simulink model "sim_IL_H2DF_2024a"  (R2024a)
settings: Solver=FixedStepAuto  StartTime=0.0  StopTime=4899  FixedStep=1  RelTol=1e-3  EnableMultiTasking=on
model workspace (MAT data in the model file):
  enable_IMEP_noise = 100
  enable_IMEP_offset = 1
values from neighbouring files (symbols this model uses):
  IL = struct()    [init_simulink_IL_H2DF.m]
undefined symbols (not defined in the file or in its folder): C2C_NMPC, cost_length, horizon_length, y_ref_buf
libraries: dspswit3 x4, deeplib x1
(part 1 of 2)
settings Model: ExtModeTrigDuration=2  Creator=maxim  LastModifiedBy=winkler_a
settings SolverCC: PositivePriorityOrder=on
settings OptimizationCC: EnhancedBackFolding=on  PassReuseOutputArgsAs=Individual arguments  ZeroExternalMemoryAtStartup=off  ZeroInternalMemoryAtStartup=off  MaxStackSize=64  OptimizeBlockOrder=speed  DifferentSizesBufferReuse=on  OptimizationCustomize=off  EfficientTunableParamExpr=on
settings DebuggingCC: ParameterTunabilityLossMsg=error
settings HardwareCC: ProdBitPerPointer=32  ProdBitPerSizeT=32  ProdBitPerPtrDiffT=32  ProdLargestAtomicInteger=Long  ProdLargestAtomicFloat=Double  ProdWordSize=32  ProdLongLongMode=on  ProdHWDeviceType=ARM Compatible->ARM Cortex
settings RTWCC: Description=Embedded Coder  SystemTargetFile=ert.tlc  HardwareBoard=Raspberry Pi  TLCOptions="-aInlineSetEventsForThisBaseRateFcn=TLC_FALSE -aSuppressMultiTaskScheduler=TLC_FALSE  -aRateBasedStepFcn=0"  TemplateMakefile=ert_default_tmf  GenerateReport=on  RTWUseSimCustomCode=on  Toolchain=GNU GCC Embedded Linux  BuildConfiguration=Faster Runs  CodeExecutionProfiling=on  GPUComputeCapability=3.5
settings CodeAppCC: ForceParamTrailComments=on  IgnoreCustomStorageClasses=off  OperatorAnnotations=on  SimulinkDataObjDesc=on  SFDataObjDesc=on  InsertBlockDesc=on
settings ERTTargetCC: SupportContinuousTime=on  SupportNonInlinedSFcns=on  SupportVariableSizeSignals=on

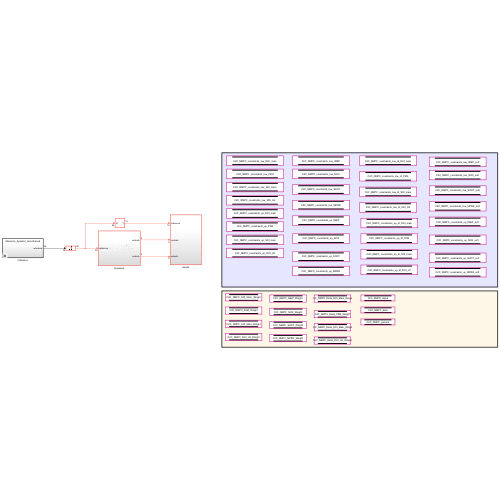
[thumbnail: Simulink's stored preview of the top-level diagram]
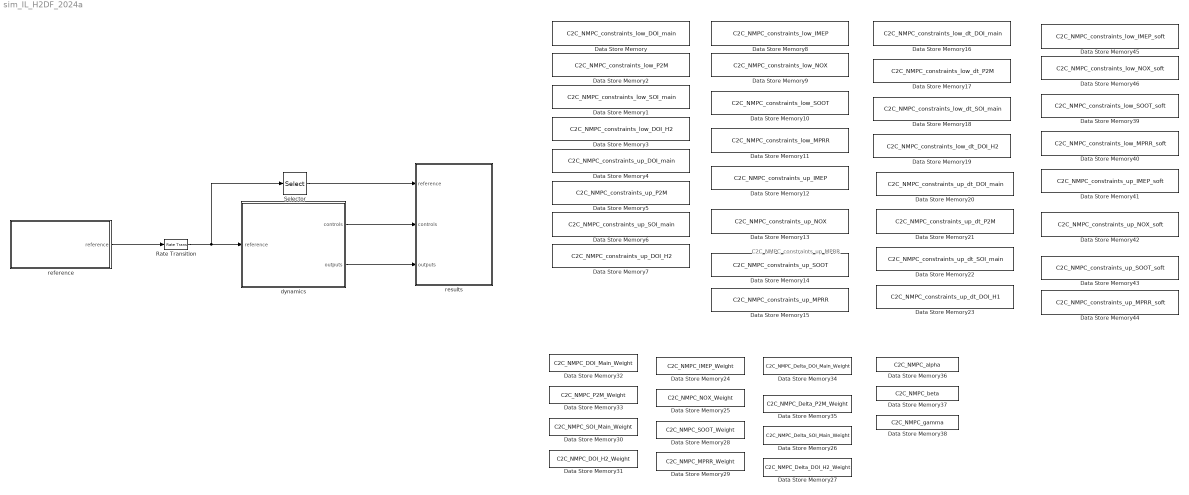
== system sim_IL_H2DF_2024a ==
  note: C2C_NMPC_constraints_up_MPRR
  Data Store Memory : DataStoreMemory  DataStoreName=C2C_NMPC_constraints_low_DOI_main  WriteAfterWriteMsg=warning  ShowAdditionalParam=off
  Data Store Memory1 : DataStoreMemory  DataStoreName=C2C_NMPC_constraints_low_SOI_main  WriteAfterWriteMsg=warning  ShowAdditionalParam=off
  Data Store Memory10 : DataStoreMemory  DataStoreName=C2C_NMPC_constraints_low_SOOT  WriteAfterWriteMsg=warning  ShowAdditionalParam=off
  Data Store Memory11 : DataStoreMemory  DataStoreName=C2C_NMPC_constraints_low_MPRR  WriteAfterWriteMsg=warning  ShowAdditionalParam=off
  Data Store Memory12 : DataStoreMemory  DataStoreName=C2C_NMPC_constraints_up_IMEP  WriteAfterWriteMsg=warning  ShowAdditionalParam=off
  Data Store Memory13 : DataStoreMemory  DataStoreName=C2C_NMPC_constraints_up_NOX  WriteAfterWriteMsg=warning  ShowAdditionalParam=off
  Data Store Memory14 : DataStoreMemory  DataStoreName=C2C_NMPC_constraints_up_SOOT  WriteAfterWriteMsg=warning  ShowAdditionalParam=off
  Data Store Memory15 : DataStoreMemory  DataStoreName=C2C_NMPC_constraints_up_MPRR  WriteAfterWriteMsg=warning  ShowAdditionalParam=off
  Data Store Memory16 : DataStoreMemory  DataStoreName=C2C_NMPC_constraints_low_dt_DOI_main  WriteAfterWriteMsg=warning  ShowAdditionalParam=off
  Data Store Memory17 : DataStoreMemory  DataStoreName=C2C_NMPC_constraints_low_dt_P2M  WriteAfterWriteMsg=warning  ShowAdditionalParam=off
  Data Store Memory18 : DataStoreMemory  DataStoreName=C2C_NMPC_constraints_low_dt_SOI_main  WriteAfterWriteMsg=warning  ShowAdditionalParam=off
  Data Store Memory19 : DataStoreMemory  DataStoreName=C2C_NMPC_constraints_low_dt_DOI_H2  WriteAfterWriteMsg=warning  ShowAdditionalParam=off
  Data Store Memory2 : DataStoreMemory  DataStoreName=C2C_NMPC_constraints_low_P2M  WriteAfterWriteMsg=warning  ShowAdditionalParam=off
  Data Store Memory20 : DataStoreMemory  DataStoreName=C2C_NMPC_constraints_up_dt_DOI_main  WriteAfterWriteMsg=warning  ShowAdditionalParam=off
  Data Store Memory21 : DataStoreMemory  DataStoreName=C2C_NMPC_constraints_up_dt_P2M  WriteAfterWriteMsg=warning  ShowAdditionalParam=off
  Data Store Memory22 : DataStoreMemory  DataStoreName=C2C_NMPC_constraints_up_dt_SOI_main  WriteAfterWriteMsg=warning  ShowAdditionalParam=off
  Data Store Memory23 : DataStoreMemory  DataStoreName=C2C_NMPC_constraints_up_dt_DOI_H1  WriteAfterWriteMsg=warning  ShowAdditionalParam=off
  Data Store Memory24 : DataStoreMemory  DataStoreName=C2C_NMPC_IMEP_Weight  WriteAfterWriteMsg=warning  ShowAdditionalParam=off
  Data Store Memory25 : DataStoreMemory  DataStoreName=C2C_NMPC_NOX_Weight  WriteAfterWriteMsg=warning  ShowAdditionalParam=off
  Data Store Memory26 : DataStoreMemory  DataStoreName=C2C_NMPC_Delta_SOI_Main_Weight  WriteAfterWriteMsg=warning  ShowAdditionalParam=off
  Data Store Memory27 : DataStoreMemory  DataStoreName=C2C_NMPC_Delta_DOI_H2_Weight  WriteAfterWriteMsg=warning  ShowAdditionalParam=off
  Data Store Memory28 : DataStoreMemory  DataStoreName=C2C_NMPC_SOOT_Weight  WriteAfterWriteMsg=warning  ShowAdditionalParam=off
  Data Store Memory29 : DataStoreMemory  DataStoreName=C2C_NMPC_MPRR_Weight  WriteAfterWriteMsg=warning  ShowAdditionalParam=off
  Data Store Memory3 : DataStoreMemory  DataStoreName=C2C_NMPC_constraints_low_DOI_H2  WriteAfterWriteMsg=warning  ShowAdditionalParam=off
  Data Store Memory30 : DataStoreMemory  DataStoreName=C2C_NMPC_SOI_Main_Weight  WriteAfterWriteMsg=warning  ShowAdditionalParam=off
  Data Store Memory31 : DataStoreMemory  DataStoreName=C2C_NMPC_DOI_H2_Weight  WriteAfterWriteMsg=warning  ShowAdditionalParam=off
  Data Store Memory32 : DataStoreMemory  DataStoreName=C2C_NMPC_DOI_Main_Weight  WriteAfterWriteMsg=warning  ShowAdditionalParam=off
  Data Store Memory33 : DataStoreMemory  DataStoreName=C2C_NMPC_P2M_Weight  WriteAfterWriteMsg=warning  ShowAdditionalParam=off
  Data Store Memory34 : DataStoreMemory  DataStoreName=C2C_NMPC_Delta_DOI_Main_Weight  WriteAfterWriteMsg=warning  ShowAdditionalParam=off
  Data Store Memory35 : DataStoreMemory  DataStoreName=C2C_NMPC_Delta_P2M_Weight  WriteAfterWriteMsg=warning  ShowAdditionalParam=off
  Data Store Memory36 : DataStoreMemory  DataStoreName=C2C_NMPC_alpha  WriteAfterWriteMsg=warning  ShowAdditionalParam=off
  Data Store Memory37 : DataStoreMemory  DataStoreName=C2C_NMPC_beta  WriteAfterWriteMsg=warning  ShowAdditionalParam=off
  Data Store Memory38 : DataStoreMemory  DataStoreName=C2C_NMPC_gamma  WriteAfterWriteMsg=warning  ShowAdditionalParam=off
  Data Store Memory39 : DataStoreMemory  DataStoreName=C2C_NMPC_constraints_low_SOOT_soft  WriteAfterWriteMsg=warning  ShowAdditionalParam=off
  Data Store Memory4 : DataStoreMemory  DataStoreName=C2C_NMPC_constraints_up_DOI_main  WriteAfterWriteMsg=warning  ShowAdditionalParam=off
  Data Store Memory40 : DataStoreMemory  DataStoreName=C2C_NMPC_constraints_low_MPRR_soft  WriteAfterWriteMsg=warning  ShowAdditionalParam=off
  Data Store Memory41 : DataStoreMemory  DataStoreName=C2C_NMPC_constraints_up_IMEP_soft  WriteAfterWriteMsg=warning  ShowAdditionalParam=off
  Data Store Memory42 : DataStoreMemory  DataStoreName=C2C_NMPC_constraints_up_NOX_soft  WriteAfterWriteMsg=warning  ShowAdditionalParam=off
  Data Store Memory43 : DataStoreMemory  DataStoreName=C2C_NMPC_constraints_up_SOOT_soft  WriteAfterWriteMsg=warning  ShowAdditionalParam=off
  Data Store Memory44 : DataStoreMemory  DataStoreName=C2C_NMPC_constraints_up_MPRR_soft  WriteAfterWriteMsg=warning  ShowAdditionalParam=off
  Data Store Memory45 : DataStoreMemory  DataStoreName=C2C_NMPC_constraints_low_IMEP_soft  WriteAfterWriteMsg=warning  ShowAdditionalParam=off
  Data Store Memory46 : DataStoreMemory  DataStoreName=C2C_NMPC_constraints_low_NOX_soft  WriteAfterWriteMsg=warning  ShowAdditionalParam=off
  Data Store Memory5 : DataStoreMemory  DataStoreName=C2C_NMPC_constraints_up_P2M  WriteAfterWriteMsg=warning  ShowAdditionalParam=off
  Data Store Memory6 : DataStoreMemory  DataStoreName=C2C_NMPC_constraints_up_SOI_main  WriteAfterWriteMsg=warning  ShowAdditionalParam=off
  Data Store Memory7 : DataStoreMemory  DataStoreName=C2C_NMPC_constraints_up_DOI_H2  WriteAfterWriteMsg=warning  ShowAdditionalParam=off
  Data Store Memory8 : DataStoreMemory  DataStoreName=C2C_NMPC_constraints_low_IMEP  WriteAfterWriteMsg=warning  ShowAdditionalParam=off
  Data Store Memory9 : DataStoreMemory  DataStoreName=C2C_NMPC_constraints_low_NOX  WriteAfterWriteMsg=warning  ShowAdditionalParam=off
  Rate Transition : RateTransition  Integrity=off  OutPortSampleTime=1
  Selector : Selector  InputPortWidth=C2C_NMPC.Dims.n_cost*3  IndexOptions=Index vector (dialog)  Indices=1:C2C_NMPC.Dims.n_cost  OutputSizes=1
  dynamics : Subsystem
  reference : Subsystem  Variant=on  VariantControlMode=label  VariantControl=Choice  LabelModeActiveChoice=reference_dynamic_smoothened_steps_msmtn
  results : Subsystem
  wires:
  dynamics/2(outputs) -> results/3(outputs)
  Rate Transition/1 -> dynamics/1(reference), Selector/1
  dynamics/1(controls) -> results/2(controls)
  Selector/1 -> results/1(reference)
  reference/1(reference) -> Rate Transition/1

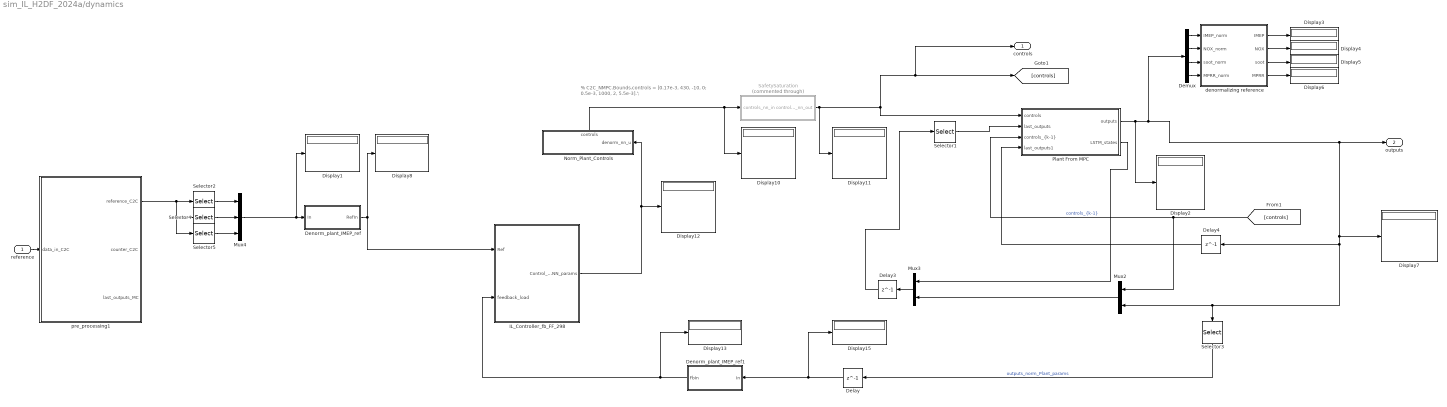
== system sim_IL_H2DF_2024a/dynamics ==
  note: % C2C_NMPC.Bounds.controls = [0.17e-3, 430, -10, 0;
      | 							0.5e-3, 1000, 2, 5.5e-3].';
  reference : Inport
  Delay : Delay  DelayLength=1  InitialCondition=0
  Delay3 : Delay  DelayLength=1  InitialCondition=C2C_NMPC.x0
  Delay4 : Delay  DelayLength=1  InitialCondition=C2C_NMPC.x0((C2C_NMPC.Dims.n_states - C2C_NMPC.Dims.n_outputs + 1):C2C_NMPC.Dims.n_states)
  Demux : Demux
  Denorm_plant_IMEP_ref : Subsystem
  Denorm_plant_IMEP_ref1 : Subsystem
  Display{1..8,10..13,15} (13 alike) : Display
  IL_Controller_fb_FF_298 : Subsystem  VariantControl=fb_LSTM_321_syn
  Mux2 : Mux  Inputs=2
  Mux3 : Mux  Inputs=2
  Mux4 : Mux  Inputs=3
  Norm_Plant_Controls : Subsystem
      settings: PortSchema="{\"entries\":[{\"content\":{\"sides\":[{\"content\":{\"connectorIds\":[\"In1\"]},\"type\":\"ConnectorPlacement.EquallySpacedRectSide\",\"uuid\":\"dacbf39b-836c-4129-b483-c12a7b9212cd\"},{\"content\":{\"side\":\"RIGHT\"},\"type\":\"ConnectorPlacement.EquallySpacedRectSide\",\"uuid\":\"2d78ef8c-cdc0-4bce-ac21-e70953625460\"},{\"content\":{\"connectorIds\":[\"Out1\"],\"side\":\"TOP\"},\"type\":\"ConnectorPlacement.EquallySpacedRectSide\",\"uuid\":\"db73efac-16fa-4395-b9f0-b65c608dd2b1\"}]},\"type\":\"ConnectorPlacement.EquallySpacedConnector\",\"uuid\":\"80b02a92-2029-43df-9a0c-0ef0e755e1ed\"}],\"packageUris\":[\"http://schema.mathworks.com/mf0/Connector/R2020b\"],\"version\":\"1.0\"}"
  Plant From MPC : Subsystem  Variant=on  VariantControlMode=label  VariantControl=Choice  LabelModeActiveChoice=Choice
  SafetySaturation : Subsystem  Commented=through
  Selector1 : Selector  IndexOptions=Index vector (dialog)  Indices=[(C2C_NMPC.Dims.n_states - C2C_NMPC.Dims.n_outputs + 1):C2C_NMPC.Dims.n_states]  OutputSizes=1
  Selector2 : Selector  IndexOptions=Index vector (dialog)  Indices=5  OutputSizes=1
  Selector3 : Selector  IndexOptions=Index vector (dialog)  Indices=[1]  OutputSizes=1
  Selector4 : Selector  IndexOptions=Index vector (dialog)  Indices=[ (C2C_NMPC.Dims.n_cost + 5) : (C2C_NMPC.Dims.n_cost + 5) ]  OutputSizes=1
  Selector5 : Selector  IndexOptions=Index vector (dialog)  Indices=[ (C2C_NMPC.Dims.n_cost * 2 + 5) : (C2C_NMPC.Dims.n_cost * 2 + 5 ) ]  OutputSizes=1
  denormalizing reference : Subsystem
  pre_processing1 : Subsystem
  controls : Outport
  outputs : Outport  Port=2
  wires:
  Delay3/1 -> Selector1/1
  Mux3/1 -> Delay3/1
  Mux2/1 -> Mux3/2
  reference/1 -> pre_processing1/1(data_in_C2C)
  Plant From MPC/1(outputs) -> outputs/1, Delay4/1, Selector3/1, Mux2/2, Display7/1, Demux/1, Display2/1
  Demux/2 -> denormalizing reference/2(NOX_norm)
  Demux/1 -> denormalizing reference/1(IMEP_norm)
  Demux/3 -> denormalizing reference/3(soot_norm)
  Demux/4 -> denormalizing reference/4(MPRR_norm)
  denormalizing reference/1(IMEP) -> Display3/1
  denormalizing reference/4(MPRR) -> Display6/1
  denormalizing reference/3(soot) -> Display5/1
  denormalizing reference/2(NOX) -> Display4/1
  IL_Controller_fb_FF_298/1(Control_norm_NN_params) -> Norm_Plant_Controls/1(denorm_nn_u), Display12/1
  Delay/1 -> Denorm_plant_IMEP_ref1/1(In), Display15/1
  Selector3/1 -> Delay/1  "outputs_norm_Plant_params"
  [controls] -> Plant From MPC/3("controls_{k-1}"), Mux2/1  "controls_{k-1}"
  Mux4/1 -> Display1/1, Denorm_plant_IMEP_ref/1(In)
  Selector2/1 -> Mux4/1
  Selector4/1 -> Mux4/2
  Selector5/1 -> Mux4/3
  pre_processing1/1(reference_C2C) -> Selector2/1, Selector4/1, Selector5/1
  Denorm_plant_IMEP_ref/1(RefIn) -> IL_Controller_fb_FF_298/1(Ref), Display8/1
  Denorm_plant_IMEP_ref1/1(FbIn) -> IL_Controller_fb_FF_298/2(feedback_load), Display13/1
  Norm_Plant_Controls/1(controls) -> Display10/1, SafetySaturation/1(controls_nn_in)
  Selector1/1 -> Plant From MPC/2(last_outputs)
  Delay4/1 -> Plant From MPC/4(last_outputs1)
  Plant From MPC/2(LSTM_states) -> Mux3/1
  SafetySaturation/1(controls_nn_out) -> Display11/1, Plant From MPC/1(controls), controls/1, [controls]

== system sim_IL_H2DF_2024a/reference ==
  note: ref is hardcoded for N=3 now
  reference_dynamic : Subsystem  Variant=on  VariantControlMode=label  VariantControl=reference_dynamic_steps  LabelModeActiveChoice=Choice_1
  reference_dynamic_constant : Subsystem  Variant=on  VariantControlMode=label  VariantControl=reference_dynamic_constant  LabelModeActiveChoice=Choice_1
  reference_dynamic_random_steps : Subsystem  Variant=on  VariantControlMode=label  VariantControl=reference_dynamic_steps_random  LabelModeActiveChoice=Choice_1
  reference_dynamic_smoothened : Subsystem  Variant=on  VariantControlMode=label  VariantControl=reference_dynamic_smoothened_steps_msmtn  LabelModeActiveChoice=Choice_1
  reference_dynamic_smoothened_random_fast_steps : Subsystem  Variant=on  VariantControlMode=label  VariantControl=reference_dynamic_smoothened_fast_steps_random  LabelModeActiveChoice=Choice_1
  reference_dynamic_smoothened_random_slow_steps : Subsystem  Variant=on  VariantControlMode=label  VariantControl=reference_dynamic_smoothened_slow_steps_random  LabelModeActiveChoice=Choice_1
  reference_static : Subsystem  VariantControl=reference_static
  reference : Outport

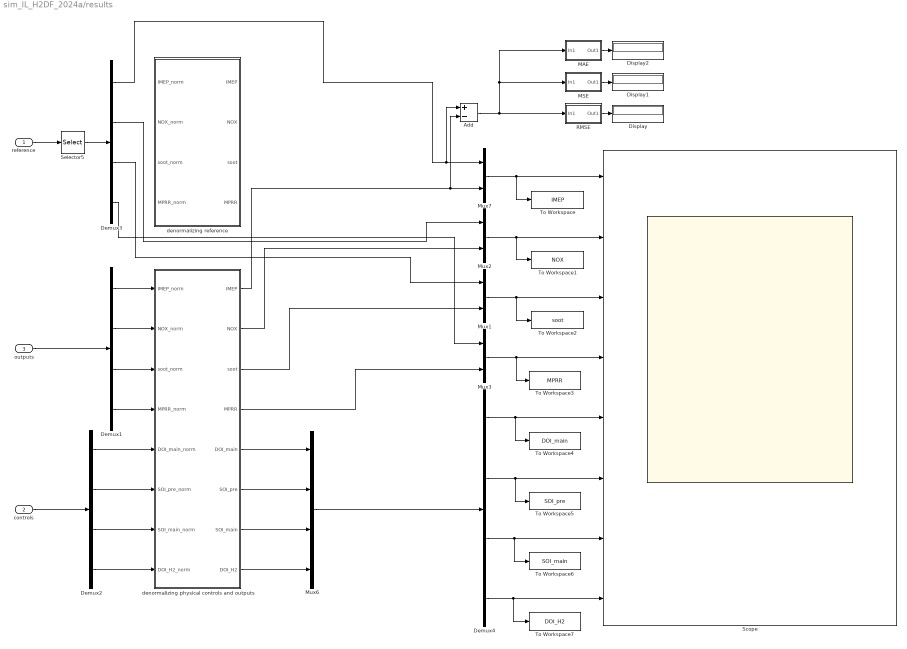
== system sim_IL_H2DF_2024a/results ==
  reference : Inport
  controls : Inport  Port=2
  outputs : Inport  Port=3
  Add : Sum  Inputs=+-
  Demux{1..4} (4 alike) : Demux
  Display : Display
  Display1 : Display
  Display2 : Display
  MAE : Subsystem
  MSE : Subsystem
  Mux{1..3,7} (4 alike) : Mux  Inputs=2
  Mux6 : Mux
  RMSE : Subsystem
  Scope : Scope  NumInputPorts=8
  Selector5 : Selector  IndexOptions=Index vector (dialog)  Indices=[(C2C_NMPC.Dims.n_controls + 1 ):(C2C_NMPC.Dims.n_cost - C2C_NMPC.Dims.n_controls)]  OutputSizes=1
  To Workspace : ToWorkspace  VariableName=IMEP  SampleTime=-1
  To Workspace1 : ToWorkspace  VariableName=NOX  SampleTime=-1
  To Workspace2 : ToWorkspace  VariableName=soot  SampleTime=-1
  To Workspace3 : ToWorkspace  VariableName=MPRR  SampleTime=-1
  To Workspace4 : ToWorkspace  VariableName=DOI_main  SampleTime=-1
  To Workspace5 : ToWorkspace  VariableName=SOI_pre  SampleTime=-1
  To Workspace6 : ToWorkspace  VariableName=SOI_main  SampleTime=-1
  To Workspace7 : ToWorkspace  VariableName=DOI_H2  SampleTime=-1
  denormalizing physical controls and outputs : Subsystem
  denormalizing reference : Subsystem
  wires:
  reference/1 -> Selector5/1
  Selector5/1 -> Demux3/1
  outputs/1 -> Demux1/1
  controls/1 -> Demux2/1
  Mux7/1 -> To Workspace/1, Scope/1
  Mux2/1 -> To Workspace1/1, Scope/2
  Demux3/1 -> Mux7/1, Add/1
  Mux3/1 -> To Workspace3/1, Scope/4
  Mux1/1 -> To Workspace2/1, Scope/3
  Demux4/2 -> To Workspace5/1, Scope/6
  Demux4/3 -> To Workspace6/1, Scope/7
  Demux4/1 -> To Workspace4/1, Scope/5
  Mux6/1 -> Demux4/1
  Demux1/1 -> denormalizing physical controls and outputs/1(IMEP_norm)
  Demux1/2 -> denormalizing physical controls and outputs/2(NOX_norm)
  Demux1/3 -> denormalizing physical controls and outputs/3(soot_norm)
  Demux1/4 -> denormalizing physical controls and outputs/4(MPRR_norm)
  Demux2/1 -> denormalizing physical controls and outputs/5(DOI_main_norm)
  Demux2/2 -> denormalizing physical controls and outputs/6(SOI_pre_norm)
  Demux2/3 -> denormalizing physical controls and outputs/7(SOI_main_norm)
  denormalizing physical controls and outputs/1(IMEP) -> Add/2, Mux7/2
  denormalizing physical controls and outputs/5(DOI_main) -> Mux6/1
  denormalizing physical controls and outputs/6(SOI_pre) -> Mux6/2
  denormalizing physical controls and outputs/7(SOI_main) -> Mux6/3
  Demux3/3 -> Mux1/1
  Demux3/4 -> Mux3/1
  denormalizing physical controls and outputs/2(NOX) -> Mux2/2
  denormalizing physical controls and outputs/3(soot) -> Mux1/2
  denormalizing physical controls and outputs/4(MPRR) -> Mux3/2
  Demux2/4 -> denormalizing physical controls and outputs/8(DOI_H2_norm)
  denormalizing physical controls and outputs/8(DOI_H2) -> Mux6/4
  Demux4/4 -> To Workspace7/1, Scope/8
  Demux3/2 -> Mux2/1
  Add/1 -> MAE/1(In1), MSE/1(In1), RMSE/1(In1)
  RMSE/1(Out1) -> Display/1
  MSE/1(Out1) -> Display1/1
  MAE/1(Out1) -> Display2/1

== system sim_IL_H2DF_2024a/dynamics/Denorm_plant_IMEP_ref ==
  In : Inport
  Constant : Constant  Value=C2C_NMPC.Normalization.outputs.mean(1)
  Gain : Gain  Gain=C2C_NMPC.Normalization.outputs.std(1)
  Sum6 : Sum  Inputs=|++
  RefIn : Outport
  wires:
  In/1 -> Gain/1  "IMEP"
  Sum6/1 -> RefIn/1
  Gain/1 -> Sum6/1
  Constant/1 -> Sum6/2

== system sim_IL_H2DF_2024a/dynamics/Denorm_plant_IMEP_ref1 ==
  In : Inport
  Constant : Constant  Value=C2C_NMPC.Normalization.outputs.mean(1)
  Gain : Gain  Gain=C2C_NMPC.Normalization.outputs.std(1)
  Sum6 : Sum  Inputs=|++
  FbIn : Outport
  wires:
  In/1 -> Gain/1  "IMEP"
  Sum6/1 -> FbIn/1
  Gain/1 -> Sum6/1
  Constant/1 -> Sum6/2

== system sim_IL_H2DF_2024a/dynamics/IL_Controller_fb_FF_298 ==
  Ref : Inport
  feedback_load : Inport  Port=2
  Data Type Conversion : DataTypeConversion  OutDataTypeStr=double  SaturateOnIntegerOverflow=off  RndMeth=Floor
  Denorm_NN_Controls : Subsystem
  Mux : Mux  Inputs=2
  Norm_NN_IMEP_ref : Subsystem
  Norm_NN_IMEP_ref1 : Subsystem
  Predict : deeplib/Predict  Network=Network from MAT-file  NetworkFunction=squeezenet  NetworkFilePath=h2df_model_2024_0012_0008_0298.mat  MiniBatchSize=512  InputDataFormats={'',''}  Predictions=on  Activations={}  ForceInterpretedSim=off  EnableDLNetwork=on  LastKnownNetworkFilePath=''  LastKnownNetworkTimeStamp=''
  Control_norm_NN_params : Outport
  wires:
  Ref/1 -> Norm_NN_IMEP_ref/1(In)
  Data Type Conversion/1 -> Denorm_NN_Controls/1(controls_nn)  "Control_norm_NN_params"
  Mux/1 -> Predict/1
  Norm_NN_IMEP_ref/1(Out) -> Mux/1
  Norm_NN_IMEP_ref1/1(Out) -> Mux/2
  Denorm_NN_Controls/1(denorm_nn_u) -> Control_norm_NN_params/1
  feedback_load/1 -> Norm_NN_IMEP_ref1/1(In)
  Predict/1 -> Data Type Conversion/1

== system sim_IL_H2DF_2024a/dynamics/Norm_Plant_Controls ==
  denorm_nn_u : Inport
  Constant10 : Constant  Value=C2C_NMPC.Normalization.controls.mean(2)
  Constant11 : Constant  Value=C2C_NMPC.Normalization.controls.mean(3)
  Constant12 : Constant  Value=C2C_NMPC.Normalization.controls.mean(4)
  Constant9 : Constant  Value=C2C_NMPC.Normalization.controls.mean(1)
  Demux : Demux
  Gain4 : Gain  Gain=1/C2C_NMPC.Normalization.controls.std(1)
  Gain5 : Gain  Gain=1/C2C_NMPC.Normalization.controls.std(2)
  Gain6 : Gain  Gain=1/C2C_NMPC.Normalization.controls.std(3)
  Gain7 : Gain  Gain=1/C2C_NMPC.Normalization.controls.std(4)
  Mux1 : Mux
  Sum{4,6..8} (4 alike) : Sum  Inputs=|+-
  controls : Outport
  wires:
  Mux1/1 -> controls/1
  denorm_nn_u/1 -> Demux/1
  Sum8/1 -> Gain7/1
  Demux/3 -> Sum7/1  "SOI_main"
  Constant12/1 -> Sum8/2
  Sum7/1 -> Gain6/1
  Constant11/1 -> Sum7/2
  Gain5/1 -> Mux1/2
  Gain4/1 -> Mux1/1
  Gain7/1 -> Mux1/4
  Demux/1 -> Sum4/1  "DOI_main"
  Constant9/1 -> Sum4/2
  Demux/2 -> Sum6/1  "SOI_pre"
  Sum4/1 -> Gain4/1
  Gain6/1 -> Mux1/3
  Constant10/1 -> Sum6/2
  Demux/4 -> Sum8/1  "DOI_H2"
  Sum6/1 -> Gain5/1

== system sim_IL_H2DF_2024a/dynamics/Plant From MPC ==
  controls : Inport
  last_outputs : Inport  Port=2
  "controls_{k-1}" : Inport  Port=3
  last_outputs1 : Inport  Port=4
  Hardcoded : Subsystem  VariantControl=Choice
  outputs : Outport
  LSTM_states : Outport  Port=2

== system sim_IL_H2DF_2024a/dynamics/SafetySaturation ==
  controls_nn_in : Inport
  Demux : Demux
  Mux : Mux
  Saturation : Saturate  UpperLimit=C2C_NMPC.Bounds.controls_norm(1,2)  LowerLimit=C2C_NMPC.Bounds.controls_norm(1,1)
  Saturation1 : Saturate  UpperLimit=C2C_NMPC.Bounds.controls_norm(2,2)  LowerLimit=C2C_NMPC.Bounds.controls_norm(2,1)
  Saturation2 : Saturate  UpperLimit=C2C_NMPC.Bounds.controls_norm(3,2)  LowerLimit=C2C_NMPC.Bounds.controls_norm(3,1)
  Saturation3 : Saturate  UpperLimit=C2C_NMPC.Bounds.controls_norm(4,2)  LowerLimit=C2C_NMPC.Bounds.controls_norm(4,1)
  controls_nn_out : Outport
  wires:
  controls_nn_in/1 -> Demux/1
  Demux/1 -> Saturation/1
  Demux/2 -> Saturation1/1
  Demux/3 -> Saturation2/1
  Demux/4 -> Saturation3/1
  Mux/1 -> controls_nn_out/1
  Saturation/1 -> Mux/1
  Saturation1/1 -> Mux/2
  Saturation2/1 -> Mux/3
  Saturation3/1 -> Mux/4

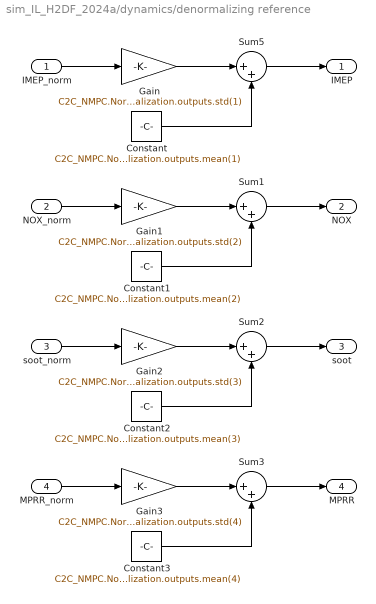
== system sim_IL_H2DF_2024a/dynamics/denormalizing reference ==
  IMEP_norm : Inport
  NOX_norm : Inport  Port=2
  soot_norm : Inport  Port=3
  MPRR_norm : Inport  Port=4
  Constant : Constant  Value=C2C_NMPC.Normalization.outputs.mean(1)
  Constant1 : Constant  Value=C2C_NMPC.Normalization.outputs.mean(2)
  Constant2 : Constant  Value=C2C_NMPC.Normalization.outputs.mean(3)
  Constant3 : Constant  Value=C2C_NMPC.Normalization.outputs.mean(4)
  Gain : Gain  Gain=C2C_NMPC.Normalization.outputs.std(1)
  Gain1 : Gain  Gain=C2C_NMPC.Normalization.outputs.std(2)
  Gain2 : Gain  Gain=C2C_NMPC.Normalization.outputs.std(3)
  Gain3 : Gain  Gain=C2C_NMPC.Normalization.outputs.std(4)
  Sum{1..3,5} (4 alike) : Sum  Inputs=|++
  IMEP : Outport
  NOX : Outport  Port=2
  soot : Outport  Port=3
  MPRR : Outport  Port=4
  wires:
  Gain/1 -> Sum5/1
  IMEP_norm/1 -> Gain/1
  Constant/1 -> Sum5/2
  Sum5/1 -> IMEP/1
  Gain1/1 -> Sum1/1
  Constant1/1 -> Sum1/2
  NOX_norm/1 -> Gain1/1
  Sum1/1 -> NOX/1
  Gain2/1 -> Sum2/1
  Constant2/1 -> Sum2/2
  soot_norm/1 -> Gain2/1
  Sum2/1 -> soot/1
  Gain3/1 -> Sum3/1
  Constant3/1 -> Sum3/2
  MPRR_norm/1 -> Gain3/1
  Sum3/1 -> MPRR/1

== system sim_IL_H2DF_2024a/dynamics/pre_processing1 ==
  data_in_C2C : Inport
  Selector : Selector  IndexOptions=Index vector (dialog)  Indices=[6]  OutputSizes=1
  normalize_last_outputs_MC : Subsystem
  normalize_reference_C2C : Subsystem
  reference_C2C : Outport  VectorParamsAs1DForOutWhenUnconnected=off
  counter_C2C : Outport  Port=2  VectorParamsAs1DForOutWhenUnconnected=off
  last_outputs_MC : Outport  Port=3  VectorParamsAs1DForOutWhenUnconnected=off
  wires:
  Selector/1 -> counter_C2C/1
  normalize_last_outputs_MC/1(last_outputs_MC) -> last_outputs_MC/1
  data_in_C2C/1 -> normalize_reference_C2C/1(data_in), normalize_last_outputs_MC/1(data_in), Selector/1
  normalize_reference_C2C/1(reference_C2C) -> reference_C2C/1

== system sim_IL_H2DF_2024a/reference/reference_dynamic ==
  reference_dynamic : Subsystem  VariantControl=Choice_1
  reference : Outport

== system sim_IL_H2DF_2024a/reference/reference_dynamic_constant ==
  reference_dynamic_constant : Subsystem  VariantControl=Choice_1
  reference : Outport

== system sim_IL_H2DF_2024a/reference/reference_dynamic_random_steps ==
  reference_dynamic_smoothened_random : Subsystem  VariantControl=Choice_1
  reference : Outport

== system sim_IL_H2DF_2024a/reference/reference_dynamic_smoothened ==
  reference_dynamic_smoothened : Subsystem  VariantControl=Choice_1
  reference : Outport

== system sim_IL_H2DF_2024a/reference/reference_dynamic_smoothened_random_fast_steps ==
  reference_dynamic_smoothened_random : Subsystem  VariantControl=Choice_1
  reference : Outport

== system sim_IL_H2DF_2024a/reference/reference_dynamic_smoothened_random_slow_steps ==
  reference_dynamic_smoothened_random : Subsystem  VariantControl=Choice_1
  reference : Outport

== system sim_IL_H2DF_2024a/reference/reference_static ==
  Add1 : Sum
  Clock : Clock
  Constant : Constant
  Constant1 : Constant  Value=[C2C_NMPC.controls_ref;C2C_NMPC.outputs_ref; zeros(C2C_NMPC.Dims.n_controls, length(C2C_NMPC.controls_ref(1, :)))]
  Mux : Mux  Inputs=3
  ref_func : MATLAB Function  TreatAsAtomicUnit=on
  reference : Outport  VectorParamsAs1DForOutWhenUnconnected=off
  wires:
  Constant1/1 -> ref_func/1(ref_norm)
  Constant/1 -> Add1/2
  Add1/1 -> ref_func/2(init_index)
  Clock/1 -> Add1/1
  Mux/1 -> reference/1
  ref_func/1(y_ref) -> Mux/3, Mux/1, Mux/2

== system sim_IL_H2DF_2024a/results/MAE ==
  In1 : Inport
  Abs : Abs  SaturateOnIntegerOverflow=off
  Add1 : Sum
  Constant : Constant  Value=4899
  Delay : Delay  DelayLength=1
  Divide : Product  Inputs=*/
  Out1 : Outport
  wires:
  Divide/1 -> Out1/1
  Add1/1 -> Delay/1
  Delay/1 -> Divide/1, Add1/2
  Abs/1 -> Add1/1
  In1/1 -> Abs/1
  Constant/1 -> Divide/2

== system sim_IL_H2DF_2024a/results/MSE ==
  In1 : Inport
  Add1 : Sum
  Constant : Constant  Value=4899
  Delay : Delay  DelayLength=1
  Divide : Product  Inputs=*/
  Square : Math  Operator=square
  Out1 : Outport
  wires:
  Divide/1 -> Out1/1
  Add1/1 -> Delay/1
  Delay/1 -> Divide/1, Add1/2
  Square/1 -> Add1/1
  In1/1 -> Square/1
  Constant/1 -> Divide/2

== system sim_IL_H2DF_2024a/results/RMSE ==
  In1 : Inport
  Add1 : Sum
  Constant : Constant  Value=4899
  Delay : Delay  DelayLength=1
  Divide : Product  Inputs=*/
  Sqrt : Sqrt
  Square : Math  Operator=square
  Out1 : Outport
  wires:
  Sqrt/1 -> Out1/1
  Add1/1 -> Delay/1
  Delay/1 -> Divide/1, Add1/2
  Square/1 -> Add1/1
  Divide/1 -> Sqrt/1
  In1/1 -> Square/1
  Constant/1 -> Divide/2

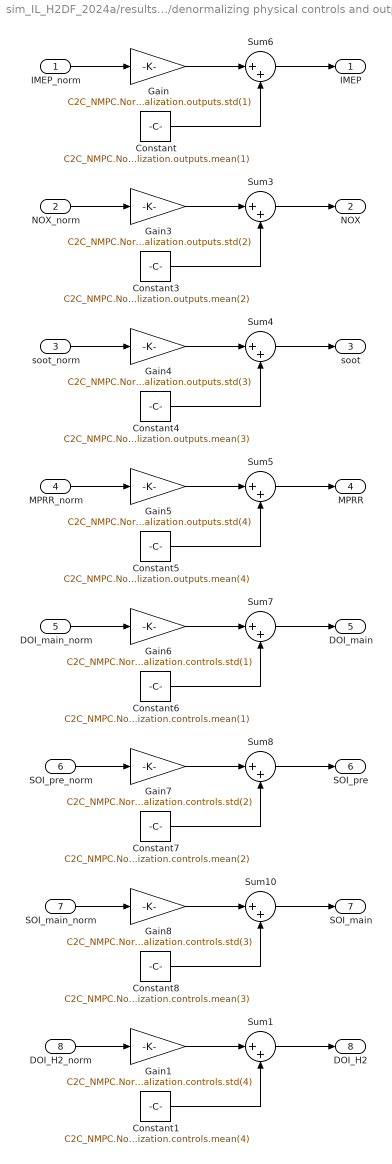
== system sim_IL_H2DF_2024a/results/denormalizing physical controls and outputs ==
  IMEP_norm : Inport
  NOX_norm : Inport  Port=2
  soot_norm : Inport  Port=3
  MPRR_norm : Inport  Port=4
  DOI_main_norm : Inport  Port=5
  SOI_pre_norm : Inport  Port=6
  SOI_main_norm : Inport  Port=7
  DOI_H2_norm : Inport  Port=8
  Constant : Constant  Value=C2C_NMPC.Normalization.outputs.mean(1)
  Constant1 : Constant  Value=C2C_NMPC.Normalization.controls.mean(4)
  Constant3 : Constant  Value=C2C_NMPC.Normalization.outputs.mean(2)
  Constant4 : Constant  Value=C2C_NMPC.Normalization.outputs.mean(3)
  Constant5 : Constant  Value=C2C_NMPC.Normalization.outputs.mean(4)
  Constant6 : Constant  Value=C2C_NMPC.Normalization.controls.mean(1)
  Constant7 : Constant  Value=C2C_NMPC.Normalization.controls.mean(2)
  Constant8 : Constant  Value=C2C_NMPC.Normalization.controls.mean(3)
  Gain : Gain  Gain=C2C_NMPC.Normalization.outputs.std(1)
  Gain1 : Gain  Gain=C2C_NMPC.Normalization.controls.std(4)
  Gain3 : Gain  Gain=C2C_NMPC.Normalization.outputs.std(2)
  Gain4 : Gain  Gain=C2C_NMPC.Normalization.outputs.std(3)
  Gain5 : Gain  Gain=C2C_NMPC.Normalization.outputs.std(4)
  Gain6 : Gain  Gain=C2C_NMPC.Normalization.controls.std(1)
  Gain7 : Gain  Gain=C2C_NMPC.Normalization.controls.std(2)
  Gain8 : Gain  Gain=C2C_NMPC.Normalization.controls.std(3)
  Sum{1,3..8,10} (8 alike) : Sum  Inputs=|++
  IMEP : Outport
  NOX : Outport  Port=2
  soot : Outport  Port=3
  MPRR : Outport  Port=4
  DOI_main : Outport  Port=5
  SOI_pre : Outport  Port=6
  SOI_main : Outport  Port=7
  DOI_H2 : Outport  Port=8
  wires:
  Gain4/1 -> Sum4/1
  Constant3/1 -> Sum3/2
  Constant4/1 -> Sum4/2
  Gain3/1 -> Sum3/1
  Constant5/1 -> Sum5/2
  Gain5/1 -> Sum5/1
  Constant/1 -> Sum6/2
  Sum3/1 -> NOX/1
  NOX_norm/1 -> Gain3/1
  Sum5/1 -> MPRR/1
  Gain/1 -> Sum6/1
  IMEP_norm/1 -> Gain/1
  Sum6/1 -> IMEP/1
  MPRR_norm/1 -> Gain5/1
  Sum4/1 -> soot/1
  soot_norm/1 -> Gain4/1
  Constant7/1 -> Sum8/2
  Gain8/1 -> Sum10/1
  Constant6/1 -> Sum7/2
  Gain7/1 -> Sum8/1
  Sum10/1 -> SOI_main/1
  DOI_main_norm/1 -> Gain6/1
  Sum7/1 -> DOI_main/1
  Gain6/1 -> Sum7/1
  Sum8/1 -> SOI_pre/1
  Constant8/1 -> Sum10/2
  SOI_main_norm/1 -> Gain8/1
  SOI_pre_norm/1 -> Gain7/1
  DOI_H2_norm/1 -> Gain1/1
  Constant1/1 -> Sum1/2
  Gain1/1 -> Sum1/1
  Sum1/1 -> DOI_H2/1

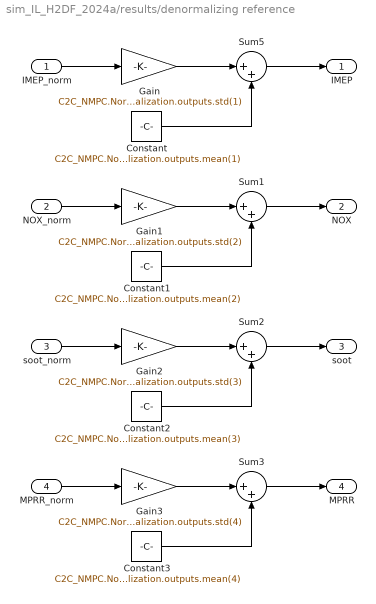
== system sim_IL_H2DF_2024a/results/denormalizing reference ==
  IMEP_norm : Inport
  NOX_norm : Inport  Port=2
  soot_norm : Inport  Port=3
  MPRR_norm : Inport  Port=4
  Constant : Constant  Value=C2C_NMPC.Normalization.outputs.mean(1)
  Constant1 : Constant  Value=C2C_NMPC.Normalization.outputs.mean(2)
  Constant2 : Constant  Value=C2C_NMPC.Normalization.outputs.mean(3)
  Constant3 : Constant  Value=C2C_NMPC.Normalization.outputs.mean(4)
  Gain : Gain  Gain=C2C_NMPC.Normalization.outputs.std(1)
  Gain1 : Gain  Gain=C2C_NMPC.Normalization.outputs.std(2)
  Gain2 : Gain  Gain=C2C_NMPC.Normalization.outputs.std(3)
  Gain3 : Gain  Gain=C2C_NMPC.Normalization.outputs.std(4)
  Sum{1..3,5} (4 alike) : Sum  Inputs=|++
  IMEP : Outport
  NOX : Outport  Port=2
  soot : Outport  Port=3
  MPRR : Outport  Port=4
  wires:
  Gain/1 -> Sum5/1
  IMEP_norm/1 -> Gain/1
  Constant/1 -> Sum5/2
  Sum5/1 -> IMEP/1
  Gain1/1 -> Sum1/1
  Constant1/1 -> Sum1/2
  NOX_norm/1 -> Gain1/1
  Sum1/1 -> NOX/1
  Gain2/1 -> Sum2/1
  Constant2/1 -> Sum2/2
  soot_norm/1 -> Gain2/1
  Sum2/1 -> soot/1
  Gain3/1 -> Sum3/1
  Constant3/1 -> Sum3/2
  MPRR_norm/1 -> Gain3/1
  Sum3/1 -> MPRR/1

== system sim_IL_H2DF_2024a/dynamics/IL_Controller_fb_FF_298/Denorm_NN_Controls ==
  controls_nn : Inport
  Constant4 : Constant  Value=IL.Normalization.outputs.mean(1)
  Constant5 : Constant  Value=IL.Normalization.outputs.mean(2)
  Constant6 : Constant  Value=IL.Normalization.outputs.mean(3)
  Constant7 : Constant  Value=IL.Normalization.outputs.mean(4)
  Demux : Demux
  Gain4 : Gain  Gain=IL.Normalization.outputs.std(1)
  Gain5 : Gain  Gain=IL.Normalization.outputs.std(2)
  Gain6 : Gain  Gain=IL.Normalization.outputs.std(3)
  Gain7 : Gain  Gain=IL.Normalization.outputs.std(4)
  Mux : Mux
  Sum{4,6..8} (4 alike) : Sum  Inputs=|++
  denorm_nn_u : Outport
  wires:
  Sum4/1 -> Mux/2
  Sum6/1 -> Mux/3
  controls_nn/1 -> Demux/1
  Demux/2 -> Gain5/1  "P2M"
  Demux/3 -> Gain6/1  "SOI_main"
  Demux/4 -> Gain7/1  "DOI_H2"
  Demux/1 -> Gain4/1  "DOI_main"
  Mux/1 -> denorm_nn_u/1
  Gain7/1 -> Sum7/1
  Gain6/1 -> Sum6/1
  Constant7/1 -> Sum7/2
  Constant5/1 -> Sum4/2
  Gain4/1 -> Sum8/1
  Gain5/1 -> Sum4/1
  Constant6/1 -> Sum6/2
  Constant4/1 -> Sum8/2
  Sum8/1 -> Mux/1
  Sum7/1 -> Mux/4

== system sim_IL_H2DF_2024a/dynamics/IL_Controller_fb_FF_298/Norm_NN_IMEP_ref ==
  In : Inport
  Constant9 : Constant  Value=IL.Normalization.inputs.mean(1)
  Gain4 : Gain  Gain=1/IL.Normalization.inputs.std(1)
  Sum4 : Sum  Inputs=|+-
  Out : Outport
  wires:
  In/1 -> Sum4/1  "IMEP"
  Constant9/1 -> Sum4/2
  Sum4/1 -> Gain4/1
  Gain4/1 -> Out/1

== system sim_IL_H2DF_2024a/dynamics/IL_Controller_fb_FF_298/Norm_NN_IMEP_ref1 ==
  In : Inport
  Constant9 : Constant  Value=IL.Normalization.inputs.mean(1)
  Gain4 : Gain  Gain=1/IL.Normalization.inputs.std(1)
  Sum4 : Sum  Inputs=|+-
  Out : Outport
  wires:
  Gain4/1 -> Out/1
  Sum4/1 -> Gain4/1
  Constant9/1 -> Sum4/2
  In/1 -> Sum4/1  "IMEP"

== system sim_IL_H2DF_2024a/dynamics/Plant From MPC/Hardcoded ==
  controls : Inport
  last_outputs : Inport  Port=2
  "controls_{k-1}" : Inport  Port=3
  last_outputs1 : Inport  Port=4
  Delay2 : Delay  DelayLength=1  InitialCondition=C2C_NMPC.x0(1:C2C_NMPC.Dims.n_LSTM_states)
  dyn_H2DF : Subsystem  Variant=on  VariantControlMode=label  VariantControl=Choice  LabelModeActiveChoice=dyn_H2DF
  dyn_H2DF_state_augmentation : Subsystem  Variant=on  VariantControlMode=label  VariantControl=Choice  LabelModeActiveChoice=dyn_H2DF
  outputs : Outport
  LSTM_states : Outport  Port=2
  wires:
  Delay2/1 -> dyn_H2DF_state_augmentation/1(last_LSTM_states), dyn_H2DF/3(last_LSTM_states)
  last_outputs/1 -> dyn_H2DF/2(last_outputs)
  dyn_H2DF_state_augmentation/1(LSTM_states) -> LSTM_states/1, Delay2/1
  controls/1 -> dyn_H2DF/1(controls)
  dyn_H2DF/1(outputs) -> outputs/1
  "controls_{k-1}"/1 -> dyn_H2DF_state_augmentation/2(controls)
  last_outputs1/1 -> dyn_H2DF_state_augmentation/3(last_outputs)

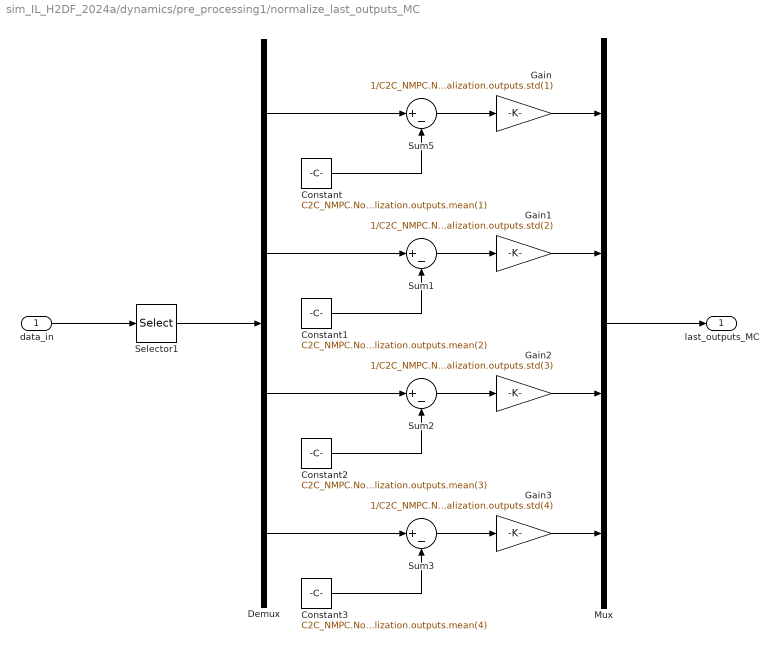
== system sim_IL_H2DF_2024a/dynamics/pre_processing1/normalize_last_outputs_MC ==
  data_in : Inport
  Constant : Constant  Value=C2C_NMPC.Normalization.outputs.mean(1)
  Constant1 : Constant  Value=C2C_NMPC.Normalization.outputs.mean(2)
  Constant2 : Constant  Value=C2C_NMPC.Normalization.outputs.mean(3)
  Constant3 : Constant  Value=C2C_NMPC.Normalization.outputs.mean(4)
  Demux : Demux
  Gain : Gain  Gain=1/C2C_NMPC.Normalization.outputs.std(1)
  Gain1 : Gain  Gain=1/C2C_NMPC.Normalization.outputs.std(2)
  Gain2 : Gain  Gain=1/C2C_NMPC.Normalization.outputs.std(3)
  Gain3 : Gain  Gain=1/C2C_NMPC.Normalization.outputs.std(4)
  Mux : Mux
  Selector1 : Selector  IndexOptions=Index vector (dialog)  Indices=[1:4]  OutputSizes=1
  Sum{1..3,5} (4 alike) : Sum  Inputs=|+-
  last_outputs_MC : Outport  VectorParamsAs1DForOutWhenUnconnected=off
  wires:
  Selector1/1 -> Demux/1
  Demux/4 -> Sum3/1
  data_in/1 -> Selector1/1
  Demux/1 -> Sum5/1
  Constant/1 -> Sum5/2
  Sum5/1 -> Gain/1
  Gain/1 -> Mux/1
  Sum3/1 -> Gain3/1
  Constant3/1 -> Sum3/2
  Mux/1 -> last_outputs_MC/1
  Gain2/1 -> Mux/3
  Demux/3 -> Sum2/1
  Constant1/1 -> Sum1/2
  Gain1/1 -> Mux/2
  Gain3/1 -> Mux/4
  Sum1/1 -> Gain1/1
  Sum2/1 -> Gain2/1
  Constant2/1 -> Sum2/2
  Demux/2 -> Sum1/1

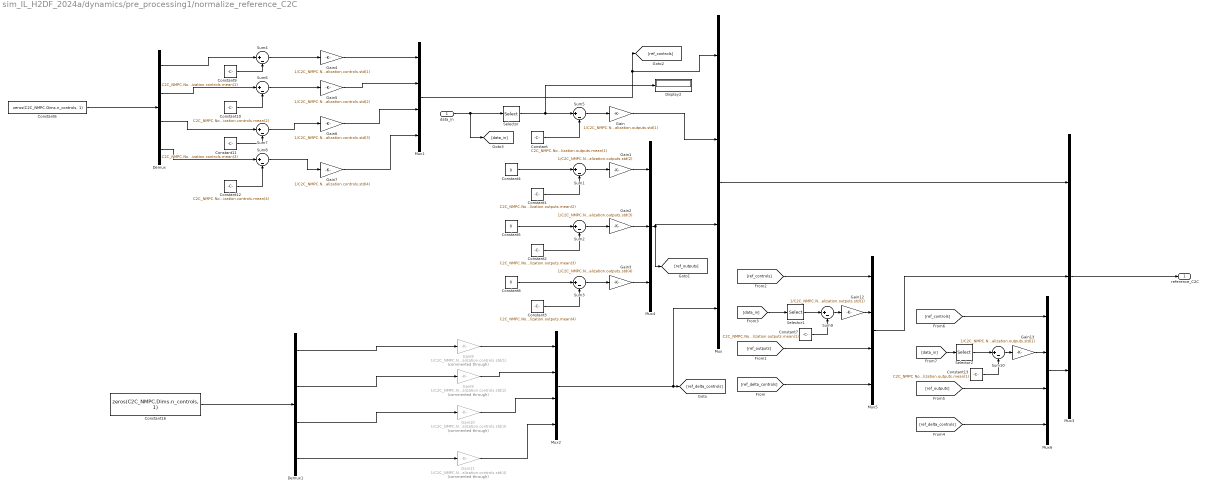
== system sim_IL_H2DF_2024a/dynamics/pre_processing1/normalize_reference_C2C ==
  data_in : Inport
  Constant : Constant  Value=C2C_NMPC.Normalization.outputs.mean(1)
  Constant1 : Constant  Value=C2C_NMPC.Normalization.outputs.mean(2)
  Constant10 : Constant  Value=C2C_NMPC.Normalization.controls.mean(2)
  Constant11 : Constant  Value=C2C_NMPC.Normalization.controls.mean(3)
  Constant12 : Constant  Value=C2C_NMPC.Normalization.controls.mean(4)
  Constant13 : Constant  Value=C2C_NMPC.Normalization.outputs.mean(1)
  Constant16 : Constant  Value=zeros(C2C_NMPC.Dims.n_controls, 1)
  Constant2 : Constant  Value=C2C_NMPC.Normalization.outputs.mean(3)
  Constant3 : Constant  Value=C2C_NMPC.Normalization.outputs.mean(4)
  Constant4 : Constant  Value=0
  Constant5 : Constant  Value=0
  Constant6 : Constant  Value=zeros(C2C_NMPC.Dims.n_controls, 1)
  Constant7 : Constant  Value=C2C_NMPC.Normalization.outputs.mean(1)
  Constant8 : Constant  Value=0
  Constant9 : Constant  Value=C2C_NMPC.Normalization.controls.mean(1)
  Demux : Demux
  Demux1 : Demux
  Display2 : Display
  Gain : Gain  Gain=1/C2C_NMPC.Normalization.outputs.std(1)
  Gain1 : Gain  Gain=1/C2C_NMPC.Normalization.outputs.std(2)
  Gain10 : Gain  Commented=through  Gain=1/C2C_NMPC.Normalization.controls.std(3)
  Gain11 : Gain  Commented=through  Gain=1/C2C_NMPC.Normalization.controls.std(4)
  Gain12 : Gain  Gain=1/C2C_NMPC.Normalization.outputs.std(1)
  Gain13 : Gain  Gain=1/C2C_NMPC.Normalization.outputs.std(1)
  Gain2 : Gain  Gain=1/C2C_NMPC.Normalization.outputs.std(3)
  Gain3 : Gain  Gain=1/C2C_NMPC.Normalization.outputs.std(4)
  Gain4 : Gain  Gain=1/C2C_NMPC.Normalization.controls.std(1)
  Gain5 : Gain  Gain=1/C2C_NMPC.Normalization.controls.std(2)
  Gain6 : Gain  Gain=1/C2C_NMPC.Normalization.controls.std(3)
  Gain7 : Gain  Gain=1/C2C_NMPC.Normalization.controls.std(4)
  Gain8 : Gain  Commented=through  Gain=1/C2C_NMPC.Normalization.controls.std(1)
  Gain9 : Gain  Commented=through  Gain=1/C2C_NMPC.Normalization.controls.std(2)
  Mux{,1..2,5..6} (5 alike) : Mux
  Mux3 : Mux  Inputs=3
  Mux4 : Mux  Inputs=3
  Selector : Selector  IndexOptions=Index vector (dialog)  Indices=[5]  OutputSizes=1
  Selector1 : Selector  IndexOptions=Index vector (dialog)  Indices=[C2C_NMPC.Dims.n_cost+5]  OutputSizes=1
  Selector2 : Selector  IndexOptions=Index vector (dialog)  Indices=[(C2C_NMPC.Dims.n_cost*2)+5]  OutputSizes=1
  Sum{1..10} (10 alike) : Sum  Inputs=|+-
  reference_C2C : Outport  VectorParamsAs1DForOutWhenUnconnected=off
  wires:
  Gain13/1 -> Mux6/2
  Selector2/1 -> Sum10/1
  Sum10/1 -> Gain13/1
  Constant13/1 -> Sum10/2
  Gain12/1 -> Mux5/2
  Constant7/1 -> Sum9/2
  Sum9/1 -> Gain12/1
  Selector1/1 -> Sum9/1
  Mux6/1 -> Mux3/3
  [ref_delta_controls] -> Mux6/4
  [ref_outputs] -> Mux6/3
  [ref_controls] -> Mux6/1
  [data_in] -> Selector2/1
  Mux5/1 -> Mux3/2
  [data_in] -> Selector1/1
  [ref_controls] -> Mux5/1
  Mux1/1 -> Mux/1, [ref_controls]
  [ref_outputs] -> Mux5/3
  [ref_delta_controls] -> Mux5/4
  Mux4/1 -> [ref_outputs], Mux/3
  Gain/1 -> Mux/2
  Gain3/1 -> Mux4/3
  Gain2/1 -> Mux4/2
  Gain1/1 -> Mux4/1
  Mux/1 -> Mux3/1
  Mux3/1 -> reference_C2C/1
  Mux2/1 -> Mux/4, [ref_delta_controls]
  Demux1/1 -> Gain8/1
  Demux1/2 -> Gain9/1
  Demux1/3 -> Gain10/1
  Demux1/4 -> Gain11/1
  Gain10/1 -> Mux2/3
  Gain8/1 -> Mux2/1
  Constant16/1 -> Demux1/1
  Gain11/1 -> Mux2/4
  Gain9/1 -> Mux2/2
  Gain6/1 -> Mux1/3
  Gain7/1 -> Mux1/4
  Demux/4 -> Sum8/1
  Sum8/1 -> Gain7/1
  Constant12/1 -> Sum8/2
  Demux/3 -> Sum7/1
  Constant11/1 -> Sum7/2
  Sum7/1 -> Gain6/1
  Gain4/1 -> Mux1/1
  Gain5/1 -> Mux1/2
  Sum6/1 -> Gain5/1
  Constant10/1 -> Sum6/2
  Demux/2 -> Sum6/1
  Constant6/1 -> Demux/1
  Constant9/1 -> Sum4/2
  Sum4/1 -> Gain4/1
  Demux/1 -> Sum4/1
  Constant3/1 -> Sum3/2
  Sum3/1 -> Gain3/1
  Constant8/1 -> Sum3/1
  Constant2/1 -> Sum2/2
  Sum2/1 -> Gain2/1
  Constant5/1 -> Sum2/1
  Constant1/1 -> Sum1/2
  Sum1/1 -> Gain1/1
  Constant4/1 -> Sum1/1
  Selector/1 -> Sum5/1, Display2/1
  Sum5/1 -> Gain/1
  data_in/1 -> Selector/1, [data_in]
  Constant/1 -> Sum5/2

== system sim_IL_H2DF_2024a/reference/reference_dynamic/reference_dynamic ==
  note: 1 -4: 0
      | 5: IMEP_ref0
      | 6 - 12: 0
      |
      | 13 - 17: 0
      | 18: IMEP_ref0
      | 19 - 24: 0
      |
      | 25 - 29: 0
      | 5: IMEP_ref0
      | 6 - 12: 0
  note: init of delays = 4 bar!
  Add1 : Sum
  Clock : Clock
  Constant : Constant
  Constant1 : Constant  Value=[C2C_NMPC.controls_ref;C2C_NMPC.outputs_ref; zeros(C2C_NMPC.Dims.n_controls, length(C2C_NMPC.controls_ref(1, :)))]
  Constant2 : Constant  Commented=on  Value=zeros(4,1)
  Constant3 : Constant  Commented=on  Value=zeros(7,1)
  Counter : dspswit3/Counter  Commented=on  Direction=Up  CountEvent=Free running  CounterSize=16 bits  MaxCount=255  InitialCount=0  Output=Count and Hit  HitValue=32  ResetInput=on  SamplesPerFrame=1  Ts=-1  CntDtype=double  HitDtype=Logical
  Delay : Delay  Commented=on  DelayLength=1
  Delay1 : Delay  Commented=on  DelayLength=1  InitialCondition=4
  Delay2 : Delay  Commented=on  InitialCondition=4
  Enabled Subsystem : Subsystem  Commented=on  TreatAsAtomicUnit=on
  GreaterThan : RelationalOperator  Commented=on  Operator=>  OutDataTypeStr=boolean  RndMeth=Simplest  InputSameDT=off
  Mux1 : Mux  Commented=on  Inputs=3
  Rate Limiter : RateLimiter  Commented=on  RisingSlewLimit=0.33  FallingSlewLimit=-0.33  SampleTimeMode=inherited  InitialCondition=3
  Signal Conversion : SignalConversion  Commented=on  OverrideOpt=off
  ref_func : MATLAB Function  InitFcn=|  TreatAsAtomicUnit=on
      | cost_length = C2C_NMPC.Dims.n_cost ;
      | horizon_length = 3;
      | %C2C_NMPC.Opts.N; 
      | y_ref_buf = zeros(cost_length, horizon_length);
  reference : Outport  VectorParamsAs1DForOutWhenUnconnected=off
  wires:
  Clock/1 -> Add1/1
  Add1/1 -> ref_func/2(init_index)
  Constant/1 -> Add1/2
  Constant1/1 -> ref_func/1(ref_norm)
  ref_func/1(y_ref) -> reference/1
  ? -> Rate Limiter/1
  Delay/1 -> Counter/1, Enabled Subsystem/Enable
  Enabled Subsystem/2(freq) -> GreaterThan/2
  GreaterThan/1 -> Delay/1
  Counter/1 -> GreaterThan/1
  Delay2/1 -> Mux1/2
  Enabled Subsystem/1(num) -> Delay1/1, Signal Conversion/1, Delay2/1
  Delay1/1 -> ?
  Signal Conversion/1 -> ?
  Constant2/1 -> Mux1/1
  Constant3/1 -> Mux1/3

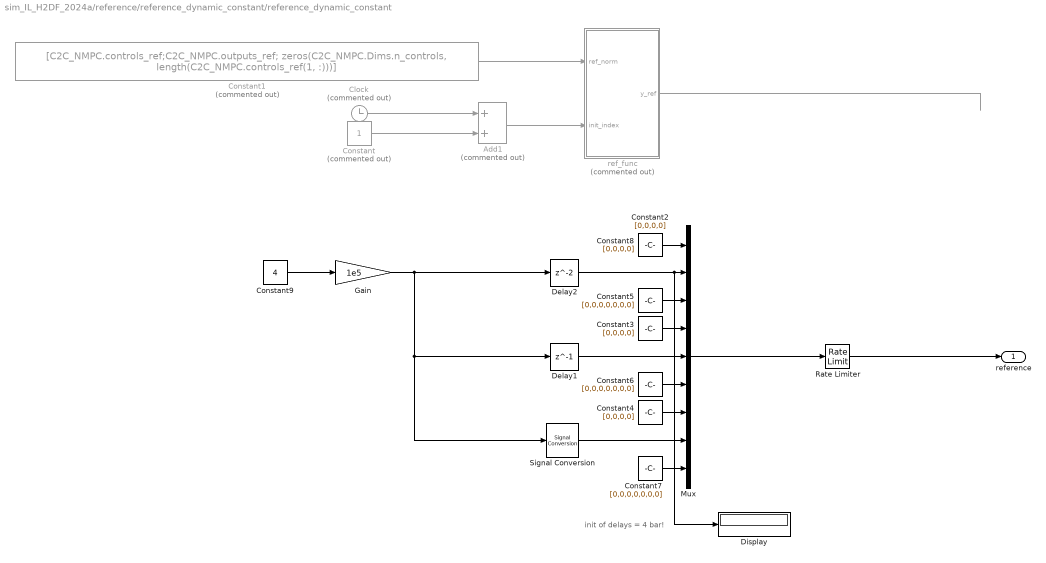
== system sim_IL_H2DF_2024a/reference/reference_dynamic_constant/reference_dynamic_constant ==
  note: init of delays = 4 bar!
  Add1 : Sum  Commented=on
  Clock : Clock  Commented=on
  Constant : Constant  Commented=on
  Constant1 : Constant  Commented=on  Value=[C2C_NMPC.controls_ref;C2C_NMPC.outputs_ref; zeros(C2C_NMPC.Dims.n_controls, length(C2C_NMPC.controls_ref(1, :)))]
  Constant{2..4,8} (4 alike) : Constant  Value=[0,0,0,0]
  Constant5 : Constant  Value=[0,0,0,0,0,0,0]
  Constant6 : Constant  Value=[0,0,0,0,0,0,0]
  Constant7 : Constant  Value=[0,0,0,0,0,0,0]
  Constant9 : Constant  Value=4
  Delay1 : Delay  DelayLength=1  InitialCondition=4
  Delay2 : Delay  InitialCondition=4
  Display : Display
  Gain : Gain  Gain=1e5
  Mux : Mux  Inputs=9
  Rate Limiter : RateLimiter  RisingSlewLimit=5000  FallingSlewLimit=-5000  SampleTimeMode=inherited  InitialCondition=3
  Signal Conversion : SignalConversion  OverrideOpt=off
  ref_func : MATLAB Function  Commented=on  InitFcn=|  TreatAsAtomicUnit=on
      | cost_length = C2C_NMPC.Dims.n_cost ;
      | horizon_length = 3;
      | %C2C_NMPC.Opts.N; 
      | y_ref_buf = zeros(cost_length, horizon_length);
  reference : Outport  VectorParamsAs1DForOutWhenUnconnected=off
  wires:
  Rate Limiter/1 -> reference/1
  Constant7/1 -> Mux/9
  Constant6/1 -> Mux/6
  Constant5/1 -> Mux/3
  Constant4/1 -> Mux/7
  Constant3/1 -> Mux/4
  Constant2/1 -> Mux/1
  Mux/1 -> Rate Limiter/1
  Delay2/1 -> Display/1, Mux/2
  Signal Conversion/1 -> Mux/8
  Constant9/1 -> Gain/1
  Delay1/1 -> Mux/5
  ref_func/1(y_ref) -> ?
  Constant1/1 -> ref_func/1(ref_norm)
  Constant/1 -> Add1/2
  Add1/1 -> ref_func/2(init_index)
  Clock/1 -> Add1/1
  Gain/1 -> Delay2/1, Delay1/1, Signal Conversion/1

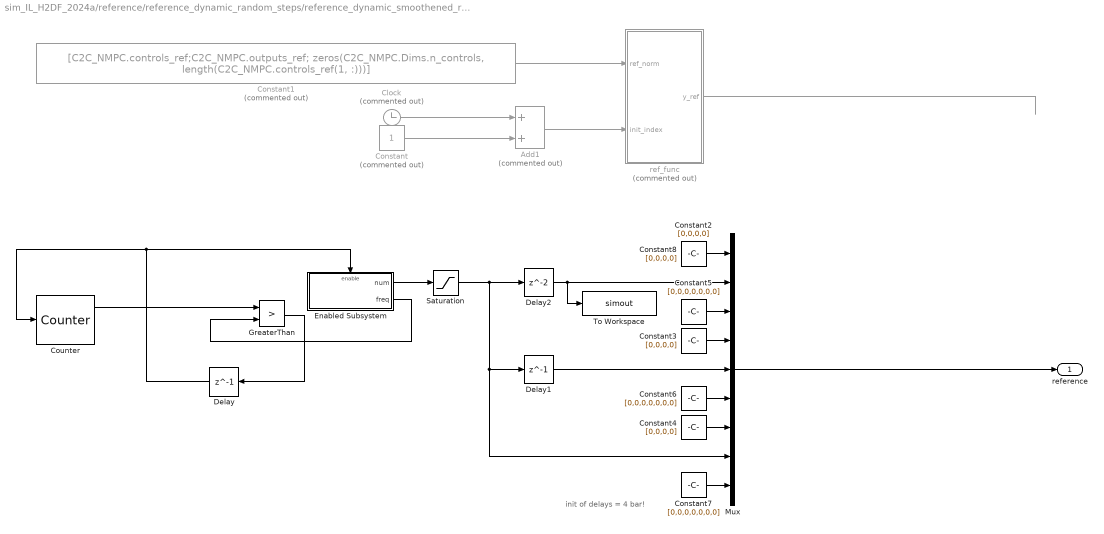
== system sim_IL_H2DF_2024a/reference/reference_dynamic_random_steps/reference_dynamic_smoothened_random ==
  note: init of delays = 4 bar!
  Add1 : Sum  Commented=on
  Clock : Clock  Commented=on
  Constant : Constant  Commented=on
  Constant1 : Constant  Commented=on  Value=[C2C_NMPC.controls_ref;C2C_NMPC.outputs_ref; zeros(C2C_NMPC.Dims.n_controls, length(C2C_NMPC.controls_ref(1, :)))]
  Constant{2..4,8} (4 alike) : Constant  Value=[0,0,0,0]
  Constant5 : Constant  Value=[0,0,0,0,0,0,0]
  Constant6 : Constant  Value=[0,0,0,0,0,0,0]
  Constant7 : Constant  Value=[0,0,0,0,0,0,0]
  Counter : dspswit3/Counter  Direction=Up  CountEvent=Free running  CounterSize=16 bits  MaxCount=255  InitialCount=0  Output=Count and Hit  HitValue=32  ResetInput=on  SamplesPerFrame=1  Ts=-1  CntDtype=double  HitDtype=Logical
  Delay : Delay  DelayLength=1
  Delay1 : Delay  DelayLength=1  InitialCondition=4*1e5
  Delay2 : Delay  InitialCondition=4*1e5
  Enabled Subsystem : Subsystem  TreatAsAtomicUnit=on
  GreaterThan : RelationalOperator  Operator=>  OutDataTypeStr=boolean  RndMeth=Simplest  InputSameDT=off
  Mux : Mux  Inputs=9
  Saturation : Saturate  UpperLimit=10*1e5  LowerLimit=4*1e5
  To Workspace : ToWorkspace  VariableName=simout  SaveFormat=Timeseries  SampleTime=-1
  ref_func : MATLAB Function  Commented=on  InitFcn=|  TreatAsAtomicUnit=on
      | cost_length = C2C_NMPC.Dims.n_cost ;
      | horizon_length = 3;
      | %C2C_NMPC.Opts.N; 
      | y_ref_buf = zeros(cost_length, horizon_length);
  reference : Outport  VectorParamsAs1DForOutWhenUnconnected=off
  wires:
  Mux/1 -> reference/1
  Constant7/1 -> Mux/9
  Constant6/1 -> Mux/6
  Constant5/1 -> Mux/3
  Constant4/1 -> Mux/7
  Constant3/1 -> Mux/4
  Constant2/1 -> Mux/1
  Delay/1 -> Counter/1, Enabled Subsystem/Enable
  Delay2/1 -> To Workspace/1, Mux/2
  Enabled Subsystem/2(freq) -> GreaterThan/2
  Counter/1 -> GreaterThan/1
  GreaterThan/1 -> Delay/1
  Delay1/1 -> Mux/5
  ref_func/1(y_ref) -> ?
  Constant1/1 -> ref_func/1(ref_norm)
  Constant/1 -> Add1/2
  Add1/1 -> ref_func/2(init_index)
  Clock/1 -> Add1/1
  Enabled Subsystem/1(num) -> Saturation/1
  Saturation/1 -> Delay2/1, Mux/8, Delay1/1

== system sim_IL_H2DF_2024a/reference/reference_dynamic_smoothened/reference_dynamic_smoothened ==
  Add1 : Sum
  Clock : Clock
  Constant : Constant
  Constant1 : Constant  Value=[IL.controls_ref;IL.outputs_ref; zeros(IL.Dims.n_outputs, length(IL.controls_ref(1, :)))]
  ref_func : MATLAB Function  InitFcn=|  TreatAsAtomicUnit=on
      | cost_length = C2C_NMPC.Dims.n_cost ;
      | horizon_length = 3;
      | %C2C_NMPC.Opts.N; 
      | y_ref_buf = zeros(cost_length, horizon_length);
  reference : Outport  VectorParamsAs1DForOutWhenUnconnected=off
  wires:
  ref_func/1(y_ref) -> reference/1
  Constant1/1 -> ref_func/1(ref_norm)
  Constant/1 -> Add1/2
  Add1/1 -> ref_func/2(init_index)
  Clock/1 -> Add1/1

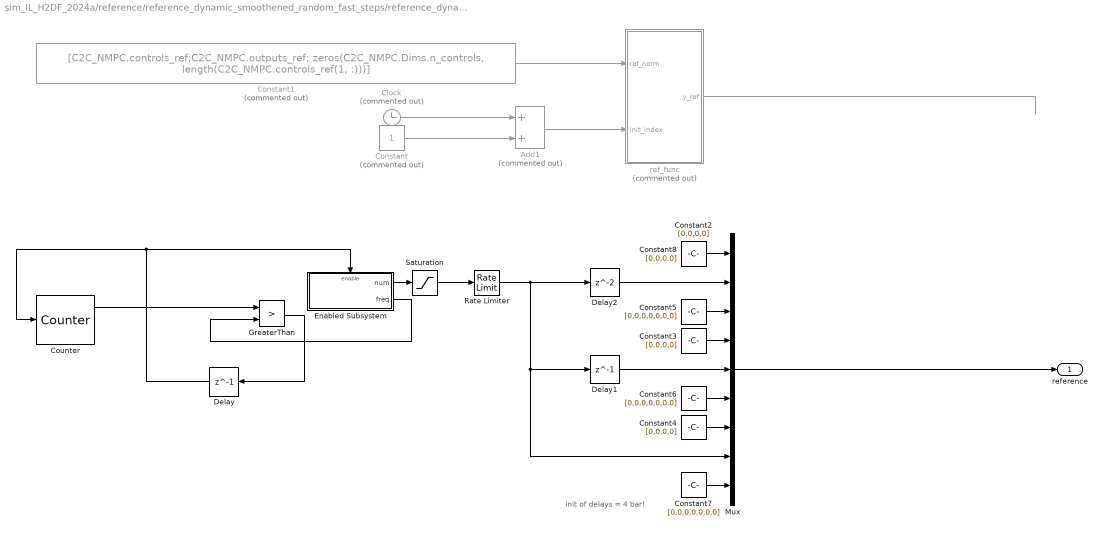
== system sim_IL_H2DF_2024a/reference/reference_dynamic_smoothened_random_fast_steps/reference_dynamic_smoothened_random ==
  note: init of delays = 4 bar!
  Add1 : Sum  Commented=on
  Clock : Clock  Commented=on
  Constant : Constant  Commented=on
  Constant1 : Constant  Commented=on  Value=[C2C_NMPC.controls_ref;C2C_NMPC.outputs_ref; zeros(C2C_NMPC.Dims.n_controls, length(C2C_NMPC.controls_ref(1, :)))]
  Constant{2..4,8} (4 alike) : Constant  Value=[0,0,0,0]
  Constant5 : Constant  Value=[0,0,0,0,0,0,0]
  Constant6 : Constant  Value=[0,0,0,0,0,0,0]
  Constant7 : Constant  Value=[0,0,0,0,0,0,0]
  Counter : dspswit3/Counter  Direction=Up  CountEvent=Free running  CounterSize=16 bits  MaxCount=255  InitialCount=0  Output=Count and Hit  HitValue=32  ResetInput=on  SamplesPerFrame=1  Ts=-1  CntDtype=double  HitDtype=Logical
  Delay : Delay  DelayLength=1
  Delay1 : Delay  DelayLength=1  InitialCondition=4*1e5
  Delay2 : Delay  InitialCondition=4*1e5
  Enabled Subsystem : Subsystem  TreatAsAtomicUnit=on
  GreaterThan : RelationalOperator  Operator=>  OutDataTypeStr=boolean  RndMeth=Simplest  InputSameDT=off
  Mux : Mux  Inputs=9
  Rate Limiter : RateLimiter  RisingSlewLimit=4000  FallingSlewLimit=-4000  SampleTimeMode=inherited  InitialCondition=4*1e5
  Saturation : Saturate  UpperLimit=10*1e5  LowerLimit=4*1e5
  ref_func : MATLAB Function  Commented=on  InitFcn=|  TreatAsAtomicUnit=on
      | cost_length = C2C_NMPC.Dims.n_cost ;
      | horizon_length = 3;
      | %C2C_NMPC.Opts.N; 
      | y_ref_buf = zeros(cost_length, horizon_length);
  reference : Outport  VectorParamsAs1DForOutWhenUnconnected=off
  wires:
  Mux/1 -> reference/1
  Constant7/1 -> Mux/9
  Constant6/1 -> Mux/6
  Constant5/1 -> Mux/3
  Constant4/1 -> Mux/7
  Constant3/1 -> Mux/4
  Constant2/1 -> Mux/1
  Delay/1 -> Counter/1, Enabled Subsystem/Enable
  Delay2/1 -> Mux/2
  Enabled Subsystem/2(freq) -> GreaterThan/2
  Counter/1 -> GreaterThan/1
  Saturation/1 -> Rate Limiter/1
  GreaterThan/1 -> Delay/1
  Enabled Subsystem/1(num) -> Saturation/1
  Delay1/1 -> Mux/5
  ref_func/1(y_ref) -> ?
  Constant1/1 -> ref_func/1(ref_norm)
  Constant/1 -> Add1/2
  Add1/1 -> ref_func/2(init_index)
  Clock/1 -> Add1/1
  Rate Limiter/1 -> Delay2/1, Mux/8, Delay1/1

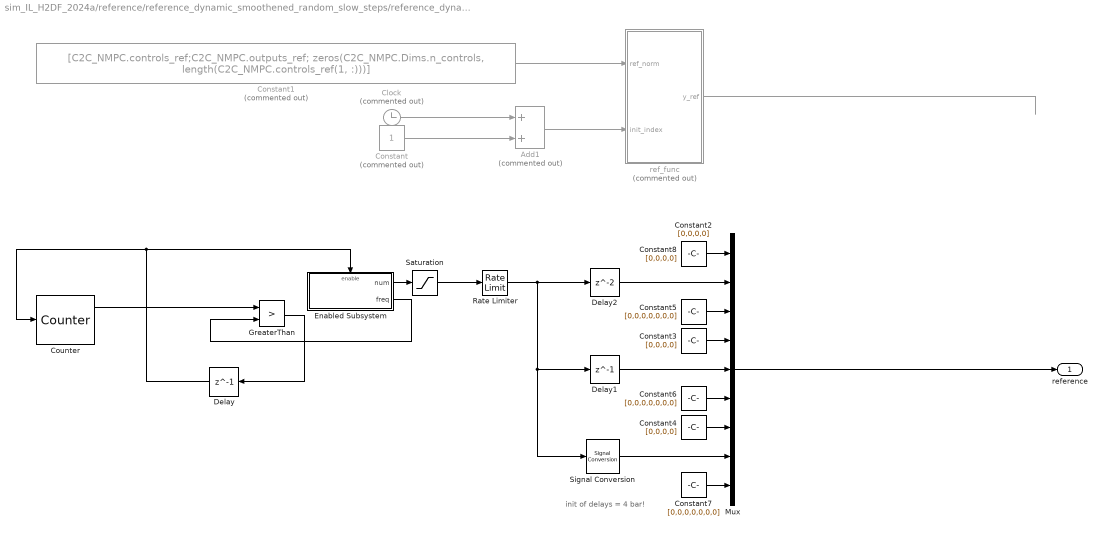
== system sim_IL_H2DF_2024a/reference/reference_dynamic_smoothened_random_slow_steps/reference_dynamic_smoothened_random ==
  note: init of delays = 4 bar!
  Add1 : Sum  Commented=on
  Clock : Clock  Commented=on
  Constant : Constant  Commented=on
  Constant1 : Constant  Commented=on  Value=[C2C_NMPC.controls_ref;C2C_NMPC.outputs_ref; zeros(C2C_NMPC.Dims.n_controls, length(C2C_NMPC.controls_ref(1, :)))]
  Constant{2..4,8} (4 alike) : Constant  Value=[0,0,0,0]
  Constant5 : Constant  Value=[0,0,0,0,0,0,0]
  Constant6 : Constant  Value=[0,0,0,0,0,0,0]
  Constant7 : Constant  Value=[0,0,0,0,0,0,0]
  Counter : dspswit3/Counter  Direction=Up  CountEvent=Free running  CounterSize=16 bits  MaxCount=255  InitialCount=0  Output=Count and Hit  HitValue=32  ResetInput=on  SamplesPerFrame=1  Ts=-1  CntDtype=double  HitDtype=Logical
  Delay : Delay  DelayLength=1
  Delay1 : Delay  DelayLength=1  InitialCondition=4*1e5
  Delay2 : Delay  InitialCondition=4*1e5
  Enabled Subsystem : Subsystem  TreatAsAtomicUnit=on
  GreaterThan : RelationalOperator  Operator=>  OutDataTypeStr=boolean  RndMeth=Simplest  InputSameDT=off
  Mux : Mux  Inputs=9
  Rate Limiter : RateLimiter  RisingSlewLimit=1500  FallingSlewLimit=-1500  SampleTimeMode=inherited  InitialCondition=4*1e5
  Saturation : Saturate  UpperLimit=10*1e5  LowerLimit=4*1e5
  Signal Conversion : SignalConversion  OverrideOpt=off
  ref_func : MATLAB Function  Commented=on  InitFcn=|  TreatAsAtomicUnit=on
      | cost_length = C2C_NMPC.Dims.n_cost ;
      | horizon_length = 3;
      | %C2C_NMPC.Opts.N; 
      | y_ref_buf = zeros(cost_length, horizon_length);
  reference : Outport  VectorParamsAs1DForOutWhenUnconnected=off
  wires:
  Mux/1 -> reference/1
  Constant7/1 -> Mux/9
  Constant6/1 -> Mux/6
  Constant5/1 -> Mux/3
  Constant4/1 -> Mux/7
  Constant3/1 -> Mux/4
  Constant2/1 -> Mux/1
  Delay/1 -> Counter/1, Enabled Subsystem/Enable
  Delay2/1 -> Mux/2
  Enabled Subsystem/2(freq) -> GreaterThan/2
  Counter/1 -> GreaterThan/1
  Signal Conversion/1 -> Mux/8
  GreaterThan/1 -> Delay/1
  Enabled Subsystem/1(num) -> Saturation/1
  Delay1/1 -> Mux/5
  ref_func/1(y_ref) -> ?
  Constant1/1 -> ref_func/1(ref_norm)
  Constant/1 -> Add1/2
  Add1/1 -> ref_func/2(init_index)
  Clock/1 -> Add1/1
  Saturation/1 -> Rate Limiter/1
  Rate Limiter/1 -> Delay2/1, Signal Conversion/1, Delay1/1

== system sim_IL_H2DF_2024a/dynamics/Plant From MPC/Hardcoded/dyn_H2DF ==
  controls : Inport  PortDimensions=C2C_NMPC.Dims.n_controls
  last_outputs : Inport  Port=2
  last_LSTM_states : Inport  Port=3
  dyn_H2DF : Subsystem  VariantControl=dyn_H2DF
  outputs : Outport

== system sim_IL_H2DF_2024a/dynamics/Plant From MPC/Hardcoded/dyn_H2DF_state_augmentation ==
  last_LSTM_states : Inport
  controls : Inport  Port=2
  last_outputs : Inport  Port=3
  dyn_H2DF_state_augmentation : Subsystem  VariantControl=dyn_H2DF
  LSTM_states : Outport

== system sim_IL_H2DF_2024a/reference/reference_dynamic/reference_dynamic/Enabled Subsystem ==
  Enable : EnablePort
  Uniform Random Number : UniformRandomNumber  Minimum=3  Maximum=8
  Uniform Random Number1 : UniformRandomNumber  Minimum=15  Maximum=150  VectorParams1D=off
  num : Outport
  freq : Outport  Port=2
  wires:
  Uniform Random Number/1 -> num/1
  Uniform Random Number1/1 -> freq/1
